simulink model "Furuta_State_Space_Simulation"  (R2020a)
settings: Solver=VariableStepAuto  StartTime=0.0  StopTime=10.0  RelTol=1e-3
values from neighbouring files (symbols this model uses):
  A = [0 1 0    0 ... (first row only)    [System_Dynamics_And_LQR_Gains.m]
  B = [0 ... (first row only)    [System_Dynamics_And_LQR_Gains.m]
  C = [ 1 0 0 0 ... (first row only)    [System_Dynamics_And_LQR_Gains.m]
  D = [ 0 ... (first row only)    [System_Dynamics_And_LQR_Gains.m]
  K = lqr(A,B,Q,R)    [System_Dynamics_And_LQR_Gains.m]
settings Model: Creator=DELL  LastModifiedBy=DELL

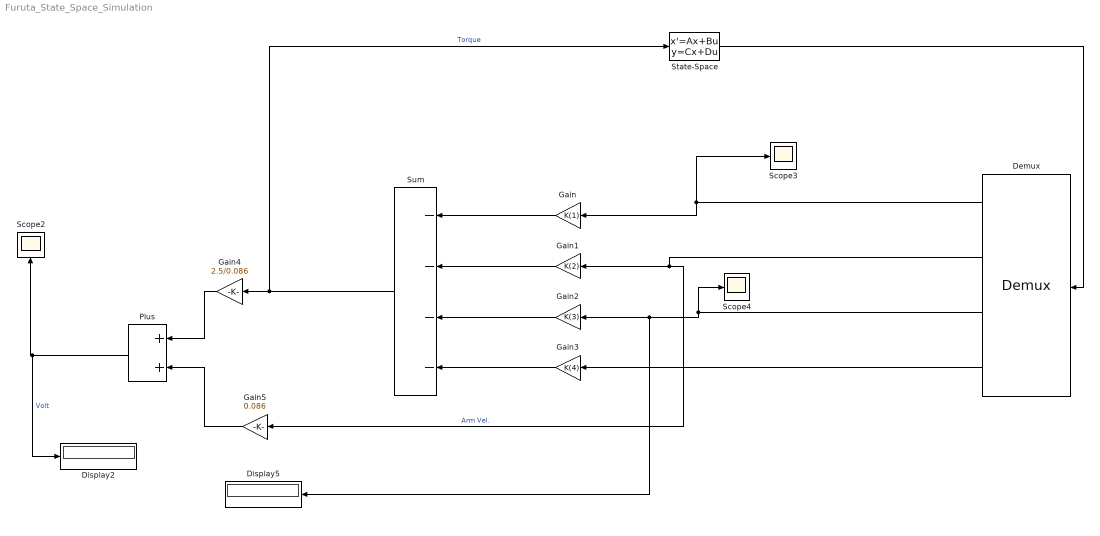
== system Furuta_State_Space_Simulation ==
  Demux : Demux
  Display2 : Display
  Display5 : Display
  Gain : Gain  Gain=K(1)
  Gain1 : Gain  Gain=K(2)
  Gain2 : Gain  Gain=K(3)
  Gain3 : Gain  Gain=K(4)
  Gain4 : Gain  Gain=2.5/0.086
  Gain5 : Gain  Gain=0.086
  Plus : Sum
  Scope2 : Scope
  Scope3 : Scope
  Scope4 : Scope
  State-Space : StateSpace  A=A  B=B  C=C  D=D  InitialCondition=[0 0 20*pi/180 0]
  Sum : Sum  Inputs=----
  wires:
  Demux/1 -> Gain/1, Scope3/1
  Sum/1 -> State-Space/1, Gain4/1  "Torque"
  Plus/1 -> Display2/1, Scope2/1  "Volt"
  Demux/2 -> Gain5/1, Gain1/1  "Arm Vel."
  Gain5/1 -> Plus/2
  Gain4/1 -> Plus/1
  Gain2/1 -> Sum/3
  Gain1/1 -> Sum/2
  Demux/4 -> Gain3/1
  Demux/3 -> Gain2/1, Display5/1, Scope4/1
  Gain3/1 -> Sum/4
  Gain/1 -> Sum/1
  State-Space/1 -> Demux/1
